simulink model "cst_robotarm_Identification"  (R2022b)
settings: Solver=ode23t  StartTime=0.0  StopTime=40  FixedStep=0.001  MaxStep=0.05  RelTol=1e-3  EnableMultiTasking=on
model workspace (MAT data in the model file):
  DCMotor_J = 0.0946866703633
  DCMotor_K = 0.477771340295
  DCMotor_Kf = 0.921434142151
  DCMotor_L = 0.000316454712175
  DCMotor_R = 4.99938152603
  Ts = 0.01
  dFilt = [1 -0.1202]
  nFilt = [0.4399 0.4399]
undefined symbols (not defined in the file or in its folder): sigbuilder_block, X, Y, Z
libraries: sm_lib x244, fl_lib x75, nesl_utility x28, ee_lib x21, simulink x6, slpidlib x6
(part 1 of 7)
settings Model: Creator=The MathWorks, Inc.  LastModifiedBy=Niki
settings SolverCC: AlgebraicLoopSolver=TrustRegion
settings DataIOCC: LimitDataPoints=on  SaveFormat=Array  InspectSignalLogs=on  SaveTime=off  ReturnWorkspaceOutputs=off
settings OptimizationCC: ExpressionDepthLimit=2147483647  LifeSpan=inf
settings DebuggingCC: UnderspecifiedInitializationDetection=Classic  MergeDetectMultiDrivingBlocksExec=none  FcnCallInpInsideContextMsg=warning  UnconnectedInputMsg=warning  UnconnectedOutputMsg=warning  UnconnectedLineMsg=warning  StateNameClashWarn=warning  SFUnexpectedBacktrackingDiag=warning  SFNoUnconditionalDefaultTransitionDiag=warning  SFExecutionAtInitializationDiag=none  SFMachineParentedDataDiag=warning  ArithmeticOperatorsInVariantConditions=warning
settings HardwareCC: ProdBitPerPointer=32  ProdBitPerSizeT=32  ProdBitPerPtrDiffT=32  ProdLargestAtomicFloat=None  ProdIntDivRoundTo=Undefined  ProdEndianess=Unspecified  ProdWordSize=32  ProdHWDeviceType=32-bit Generic
settings ModelReferenceCC: EnableRefExpFcnMdlSchedulingChecks=on  PropagateSignalLabelsOutOfModel=off
settings SFSimCC: SimUseLocalCustomCode=off  CustomCodeUndefinedFunction=UseInterfaceOnly
settings RTWCC: RTWUseLocalCustomCode=off
settings CodeAppCC: StateflowObjectComments=on
settings GRTTargetCC: TargetLangStandard=C89/C90 (ANSI)  CombineOutputUpdateFcns=off  GRTInterface=on
settings ConfigComp: CovMetricSettings=dw  CovSaveCumulativeToWorkspaceVar=on  CovSaveSingleToWorkspaceVar=on  CovExternalEMLEnable=off  CovSFcnEnable=off
settings SimscapeCC: SimscapeNormalizeSystem=off
settings ConfigurationSet: Description=SimMechanics 2G
settings DiagnosticsConfigSet: SimMechanicsUnconnectedFramePorts=none
settings ExplorerConfigSet: InternalSimMechanicsExplorerSettings="<ExplorerConfiguration><canonicalview>planar_xy</canonicalview><AnimationSetting><BasePlaybackSpeed>1.0</BasePlaybackSpeed><PlaybackSpeedFactor>1.0</PlaybackSpeedFactor></AnimationSetting><TilePanel><TileInfo><Tiles Columns=\"1\" Count=\"1\" Rows=\"1\"><Column Left=\"2\" Weight=\"1\"/><Column Left=\"708\"/><Row Top=\"2\" Weight=\"1\"/><Row Top=\"595\"/><Tile Height=\"1\" Width=\"1\" X=\"0\" Y=\"0\"/></Tiles></TileInfo><SceneInfo><SceneViewer><BGColor><R>0.80000001192092896</R><G>0.80000001192092896</G><B>0.80000001192092896</B></BGColor><Camera><Position><X>0.30752487944302698</X><Y>0.57922836563106395</Y><Z>0.35651305744246536</Z></Position><Center><X>-0.033772386749033274</X><Y>0.23793109943898419</Y><Z>0.015215791250393121</Z></Center><Up><X>-0.40824829046386307</X><Y>0.81649658092772615</Y><Z>-0.40824829046386307</Z></Up><Left>-0.063283674940751766</Left><Right>0.063283674940751766</Right><Bottom>-0.22321517040744418</Bottom><Top>0.22321517040744418</Top></Camera></SceneViewer></SceneInfo></TilePanel></ExplorerConfiguration>"

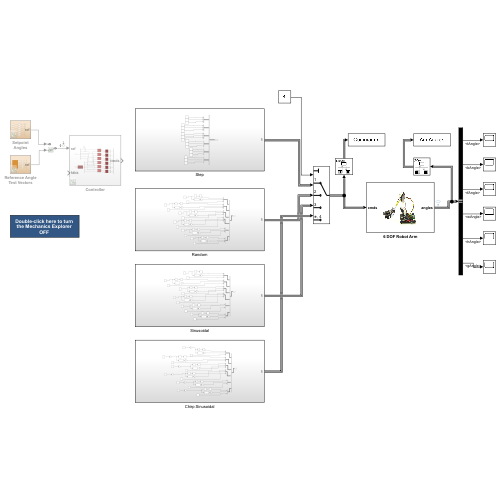
[thumbnail: Simulink's stored preview of the top-level diagram]
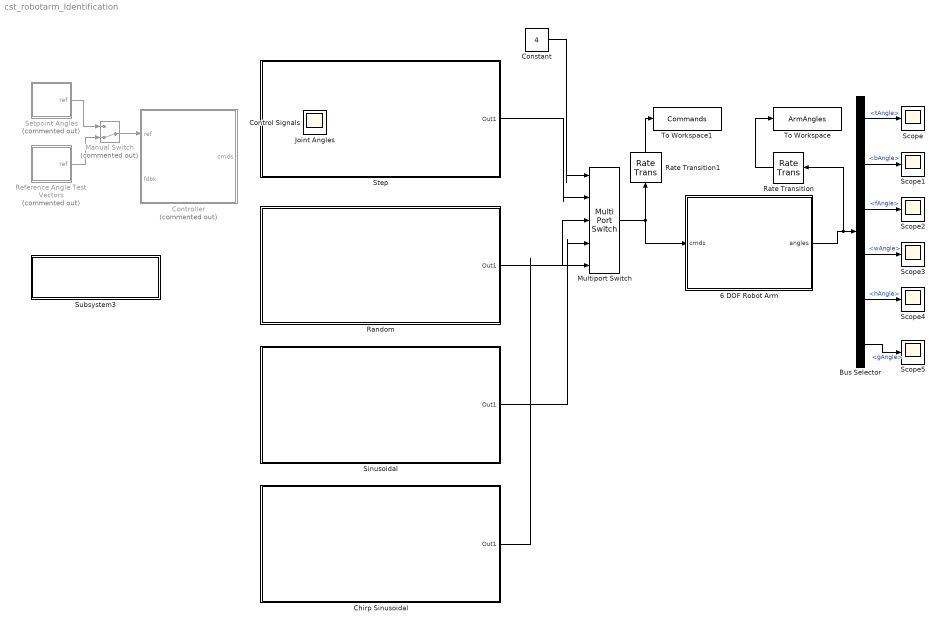
== system cst_robotarm_Identification ==
  6 DOF Robot Arm : Subsystem
      mask Display: image('RobotArmSystem.jpg',[0.2 0.05 0.6 0.9])
  Bus Selector : BusSelector  OutputSignals=tAngle,bAngle,fAngle,wAngle,hAngle,gAngle
  Chirp Sinusoidal : Subsystem
  Constant : Constant  Value=4
  Controller : Subsystem  Commented=on
  Manual Switch : ManualSwitch  Commented=on  CurrentSetting=0
  Multiport Switch : MultiPortSwitch  Inputs=4  SaturateOnIntegerOverflow=off  InputSameDT=off
  Random : Subsystem
  Rate Transition : RateTransition  OutPortSampleTime=0.01
  Rate Transition1 : RateTransition  OutPortSampleTime=0.01
  Reference Angle Test Vectors : Subsystem  Commented=on
  Scope{,1..5} (6 alike) : Scope
  Setpoint Angles : Subsystem  Commented=on
  Sinusoidal : Subsystem
  Step : Subsystem
  Subsystem3 : Subsystem
      mask init:
      | % Get current simulation mode
      | vizStatus = get_param(gcs,'SimMechanicsOpenEditorOnUpdate');
      | 
      | if strcmp(vizStatus,'on')
      |     viz = 'OFF';
      | else
      |     viz = 'ON';
      | end
      settings: OpenFcn=|
      | % Get current SimMechanics Explorer status
      | vizStatus = get_param(gcs ,'SimMechanicsOpenEditorOnUpdate');
      | 
      | if strcmp(vizStatus,'on')
      | % Set SimMechanics Explorer status to OFF
      |      set_param(gcs,'SimMechanicsOpenEditorOnUpdate','off');
      |      set_param(gcb,'BackgroundColor','[0.4706, 0.4706, 0.4706]');
      |      set_param(gcs,'SimulationCommand','update');
      | else
      | % Set SimMechanics Explorer status to ON
      |      set_param(gcs,'SimMechanicsOpenEditorOnUpdate','on');
      |      set_param(gcb,'BackgroundColor','[0.1961, 0.3412, 0.5176]')
      |      set_param(gcs,'SimulationCommand','update');
      | end
      mask Display:
      | color('white')
      | text(0.5,0.65,'Double-click here to turn\nthe Mechanics Explorer',...
      |     'horizontalAlignment','center',...
      |     'verticalAlignment','middle');
      | text(0.5,0.25,viz,...
      |     'horizontalAlignment','center',...
      |     'verticalAlignment','middle')
  To Workspace : ToWorkspace  VariableName=ArmAngles  SaveFormat=Structure With Time  SampleTime=-1
  To Workspace1 : ToWorkspace  VariableName=Commands  SaveFormat=Structure With Time  SampleTime=-1
  Control Signals : Scope
  Joint Angles : Scope
  wires:
  Manual Switch/1 -> Controller/1(ref)
  Reference Angle Test Vectors/1(ref) -> Manual Switch/2
  Setpoint Angles/1(ref) -> Manual Switch/1
  6 DOF Robot Arm/1(angles) -> Rate Transition/1, Bus Selector/1
  Bus Selector/1 -> Scope/1  "<tAngle>"
  Bus Selector/2 -> Scope1/1  "<bAngle>"
  Bus Selector/3 -> Scope2/1  "<fAngle>"
  Bus Selector/4 -> Scope3/1  "<wAngle>"
  Bus Selector/5 -> Scope4/1  "<hAngle>"
  Bus Selector/6 -> Scope5/1  "<gAngle>"
  Rate Transition/1 -> To Workspace/1
  Rate Transition1/1 -> To Workspace1/1
  Multiport Switch/1 -> 6 DOF Robot Arm/1(cmds), Rate Transition1/1
  Random/1(Out1) -> Multiport Switch/3
  Step/1(Out1) -> Multiport Switch/2
  Sinusoidal/1(Out1) -> Multiport Switch/4
  Constant/1 -> Multiport Switch/1
  Chirp Sinusoidal/1(Out1) -> Multiport Switch/5

== system cst_robotarm_Identification/6 DOF Robot Arm ==
  note: 6 DOF Robot Arm Manipulator - Electrical + Mechanical Plant Model
  cmds : Inport
  6 DOF Robot Arm Mechanics : Subsystem
      mask Display: image('RobotArm_Mechanics.jpg',[0.1 0 0.8 1])
  Bus Creator : BusCreator  Inputs=6
  Bus Selector : BusSelector  OutputSignals=tCMD,bCMD,fCMD,wCMD,hCMD,gCMD
  DC Motors : Subsystem
      mask Display: image('MultiServos.jpg',[0.25 0.1 0.5 0.8])
  PS-Simulink Converter{,1..5} (6 alike) : nesl_utility/PS-Simulink Converter  PhysicalDomain=network_engine_domain  SubClassName=ps_output  LeftPortType=input  RightPortType=output  PseudoPeriodic=off  Frequencies=[]  VectorFormat=1-D array  Unit=rad  AffineConversion=off
  angles : Outport  VectorParamsAs1DForOutWhenUnconnected=off
  wires:
  Bus Creator/1 -> angles/1
  PS-Simulink Converter2/1 -> Bus Creator/3  "fAngle"
  PS-Simulink Converter5/1 -> Bus Creator/6  "gAngle"
  PS-Simulink Converter/1 -> Bus Creator/1  "tAngle"
  PS-Simulink Converter1/1 -> Bus Creator/2  "bAngle"
  PS-Simulink Converter3/1 -> Bus Creator/4  "wAngle"
  PS-Simulink Converter4/1 -> Bus Creator/5  "hAngle"
  Bus Selector/6 -> DC Motors/6(gCMD)  "<gCMD>"
  Bus Selector/3 -> DC Motors/3(fCMD)  "<fCMD>"
  Bus Selector/4 -> DC Motors/4(wCMD)  "<wCMD>"
  Bus Selector/2 -> DC Motors/2(bCMD)  "<bCMD>"
  Bus Selector/5 -> DC Motors/5(hCMD)  "<hCMD>"
  Bus Selector/1 -> DC Motors/1(tCMD)  "<tCMD>"
  cmds/1 -> Bus Selector/1
  connections:
  PS-Simulink Converter2/LConn1 -- 6 DOF Robot Arm Mechanics/RConn3
  DC Motors/RConn7 -- 6 DOF Robot Arm Mechanics/LConn7
  DC Motors/RConn8 -- 6 DOF Robot Arm Mechanics/LConn8
  DC Motors/RConn6 -- 6 DOF Robot Arm Mechanics/LConn6
  PS-Simulink Converter/LConn1 -- 6 DOF Robot Arm Mechanics/RConn1
  DC Motors/RConn2 -- 6 DOF Robot Arm Mechanics/LConn2
  DC Motors/RConn5 -- 6 DOF Robot Arm Mechanics/LConn5
  DC Motors/RConn11 -- 6 DOF Robot Arm Mechanics/LConn11
  DC Motors/RConn12 -- 6 DOF Robot Arm Mechanics/LConn12
  DC Motors/RConn9 -- 6 DOF Robot Arm Mechanics/LConn9
  DC Motors/RConn3 -- 6 DOF Robot Arm Mechanics/LConn3
  DC Motors/RConn4 -- 6 DOF Robot Arm Mechanics/LConn4
  PS-Simulink Converter1/LConn1 -- 6 DOF Robot Arm Mechanics/RConn2
  PS-Simulink Converter4/LConn1 -- 6 DOF Robot Arm Mechanics/RConn5
  6 DOF Robot Arm Mechanics/RConn6 -- PS-Simulink Converter5/LConn1
  6 DOF Robot Arm Mechanics/RConn4 -- PS-Simulink Converter3/LConn1
  DC Motors/RConn10 -- 6 DOF Robot Arm Mechanics/LConn10
  DC Motors/RConn1 -- 6 DOF Robot Arm Mechanics/LConn1

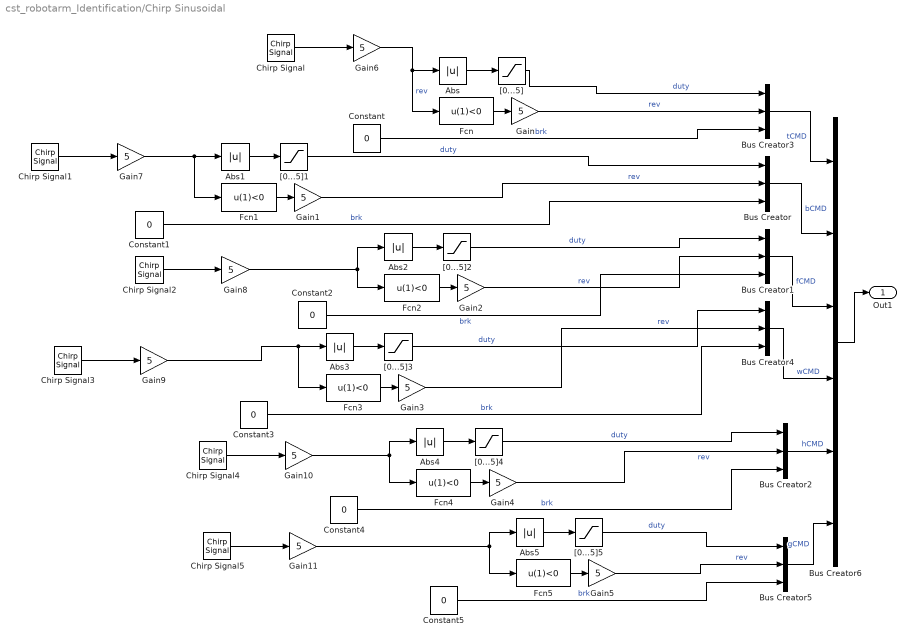
== system cst_robotarm_Identification/Chirp Sinusoidal ==
  Abs{,1..5} (6 alike) : Abs  SaturateOnIntegerOverflow=off
  Bus Creator{,1..5} (6 alike) : BusCreator  Inputs=3
  Bus Creator6 : BusCreator  Inputs=6
  Chirp Signal{,1..5} (6 alike) : simulink/Sources/Chirp Signal  f1=0.1  T=20  f2=2
  Constant{,1..5} (6 alike) : Constant  Value=0
  Fcn{,1..5} (6 alike) : Fcn  Expr=u(1)<0
  Gain{,1..11} (12 alike) : Gain  Gain=5
  [0...5]{,1..5} (6 alike) : Saturate  UpperLimit=5  LowerLimit=0
  Out1 : Outport
  wires:
  Fcn5/1 -> Gain5/1
  Gain11/1 -> Fcn5/1, Abs5/1
  Abs5/1 -> "[0...5]5"/1
  Fcn4/1 -> Gain4/1
  Gain10/1 -> Fcn4/1, Abs4/1
  Abs4/1 -> "[0...5]4"/1
  Fcn3/1 -> Gain3/1
  Gain9/1 -> Abs3/1, Fcn3/1
  Abs3/1 -> "[0...5]3"/1
  Fcn2/1 -> Gain2/1
  Gain8/1 -> Abs2/1, Fcn2/1
  Abs2/1 -> "[0...5]2"/1
  Gain7/1 -> Abs1/1, Fcn1/1
  Fcn1/1 -> Gain1/1
  Abs1/1 -> "[0...5]1"/1
  Abs/1 -> "[0...5]"/1
  Fcn/1 -> Gain/1
  Chirp Signal/1 -> Gain6/1
  Bus Creator6/1 -> Out1/1
  "[0...5]5"/1 -> Bus Creator5/1  "duty"
  Constant5/1 -> Bus Creator5/3  "brk"
  Bus Creator/1 -> Bus Creator6/2  "bCMD"
  Gain5/1 -> Bus Creator5/2  "rev"
  Bus Creator1/1 -> Bus Creator6/3  "fCMD"
  Constant3/1 -> Bus Creator4/3  "brk"
  Bus Creator5/1 -> Bus Creator6/6  "gCMD"
  Gain3/1 -> Bus Creator4/2  "rev"
  Bus Creator2/1 -> Bus Creator6/5  "hCMD"
  "[0...5]"/1 -> Bus Creator3/1  "duty"
  Bus Creator4/1 -> Bus Creator6/4  "wCMD"
  "[0...5]1"/1 -> Bus Creator/1  "duty"
  Constant1/1 -> Bus Creator/3  "brk"
  Gain1/1 -> Bus Creator/2  "rev"
  Gain2/1 -> Bus Creator1/2  "rev"
  Constant2/1 -> Bus Creator1/3  "brk"
  Constant/1 -> Bus Creator3/3  "brk"
  "[0...5]2"/1 -> Bus Creator1/1  "duty"
  Gain/1 -> Bus Creator3/2  "rev"
  Gain4/1 -> Bus Creator2/2  "rev"
  "[0...5]3"/1 -> Bus Creator4/1  "duty"
  Bus Creator3/1 -> Bus Creator6/1  "tCMD"
  "[0...5]4"/1 -> Bus Creator2/1  "duty"
  Constant4/1 -> Bus Creator2/3  "brk"
  Gain6/1 -> Abs/1, Fcn/1  "rev"
  Chirp Signal1/1 -> Gain7/1
  Chirp Signal2/1 -> Gain8/1
  Chirp Signal3/1 -> Gain9/1
  Chirp Signal4/1 -> Gain10/1
  Chirp Signal5/1 -> Gain11/1

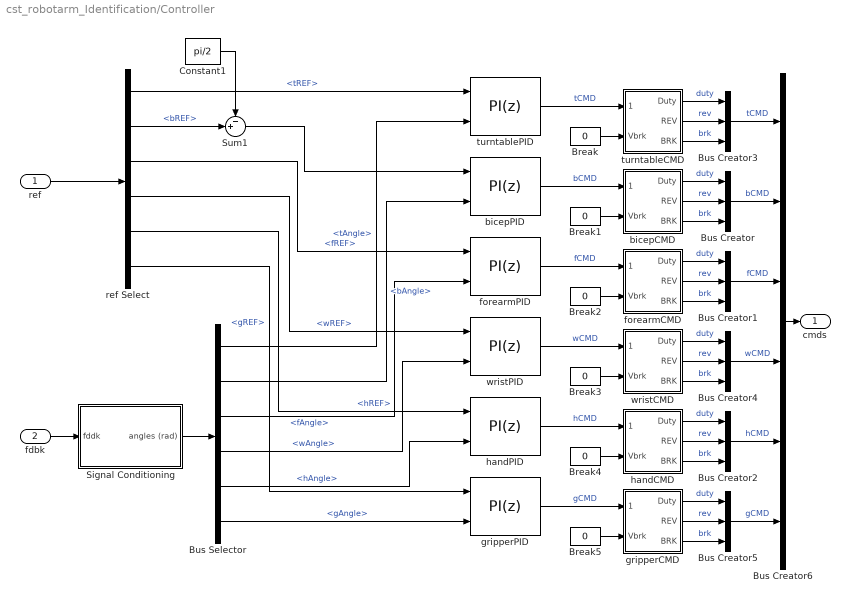
== system cst_robotarm_Identification/Controller ==
  ref : Inport
  fdbk : Inport  Port=2
  Break{,1..5} (6 alike) : Constant  Value=0
  Bus Creator{,1..5} (6 alike) : BusCreator  Inputs=3
  Bus Creator6 : BusCreator  Inputs=6
  Bus Selector : BusSelector  OutputSignals=tAngle,bAngle,fAngle,wAngle,hAngle,gAngle
  Constant1 : Constant  Value=pi/2
  Signal Conditioning : Subsystem
  Sum1 : Sum  Inputs=-+|
  bicepCMD : Subsystem
  bicepPID : slpidlib/PID Controller (2DOF)  Controller=PI  Form=Parallel  TimeDomain=Discrete-time  UseExternalTs=off  SampleTime=Ts  IntegratorMethod=Forward Euler  FilterMethod=Backward Euler  ControllerParametersSource=internal  P=17.1497999260389  I=18.7242369753632  UseKiTs=off  D=2.0  N=25  UseFilter=on  b=0.317016964341213  c=1  TunerSelectOption=Transfer Function Based (PID Tuner App)  InitialConditionSource=internal  InitialConditionForIntegrator=0  InitialConditionForFilter=0  DifferentiatorICPrevScaledInput=0  ExternalReset=none  TrackingMode=off  Kt=1  LimitOutput=on  SatLimitsSource=internal  UpperSaturationLimit=5  LowerSaturationLimit=-5  LinearizeAsGain=on  AntiWindupMode=clamping  Kb=1  LimitIntegrator=off  UpperIntegratorSaturationLimit=inf  LowerIntegratorSaturationLimit=-inf  POutMin=[]  POutMax=[]  IOutMin=[]  IOutMax=[]  DOutMin=[]  DOutMax=[]  NOutMin=[]  NOutMax=[]  bOutMin=[]  bOutMax=[]  cOutMin=[]  cOutMax=[]  SumOutMin=[]  SumOutMax=[]  SaturationOutMin=[]  SaturationOutMax=[]  PParamMin=[]  PParamMax=[]  IParamMin=[]  IParamMax=[]  DParamMin=[]  DParamMax=[]  NParamMin=[]  NParamMax=[]  bParamMin=[]  bParamMax=[]  cParamMin=[]  cParamMax=[]  KbParamMin=[]  KbParamMax=[]  KtParamMin=[]  KtParamMax=[]  KbOutMin=[]  KbOutMax=[]  KtOutMin=[]  KtOutMax=[]  IntegratorOutMin=[]  IntegratorOutMax=[]  FilterOutMin=[]  FilterOutMax=[]  SumI1OutMin=[]  SumI1OutMax=[]  SumI2OutMin=[]  SumI2OutMax=[]  SumI3OutMin=[]  SumI3OutMax=[]  SumI4OutMin=[]  SumI4OutMax=[]  SumDOutMin=[]  SumDOutMax=[]  Sum1OutMin=[]  Sum1OutMax=[]  Sum2OutMin=[]  Sum2OutMax=[]  Sum3OutMin=[]  Sum3OutMax=[]  DifferentiatorOutMin=[]  DifferentiatorOutMax=[]  FilterDiffOutCoefMin=[]  FilterDiffOutCoefMax=[]  ReciprocalOutMin=[]  ReciprocalOutMax=[]  SumDenOutMin=[]  SumDenOutMax=[]  SumNumOutMin=[]  SumNumOutMax=[]  DivideOutMin=[]  DivideOutMax=[]  UdiffTsProdOutMin=[]  UdiffTsProdOutMax=[]  NTsProdOutMin=[]  NTsProdOutMax=[]  UintegralTsProdOutMin=[]  UintegralTsProdOutMax=[]  UngainTsProdOutMin=[]  UngainTsProdOutMax=[]  ClampingZeroOutDataTypeStr=Inherit: Inherit via back propagation  ClampingZeroOutMin=[]  ClampingZeroOutMax=[]  FilterDenConstantOutDataTypeStr=Inherit: Inherit via back propagation  FilterDenConstantOutMin=[]  FilterDenConstantOutMax=[]  PCopyOutDataTypeStr=Inherit: Inherit via back propagation  PCopyOutMin=[]  PCopyOutMax=[]  NCopyOutDataTypeStr=Inherit: Inherit via back propagation  NCopyOutMin=[]  NCopyOutMax=[]  IntegratorContinuousStateAttributes=''  IntegratorStateMustResolveToSignalObject=off  IntegratorRTWStateStorageClass=Auto  FilterContinuousStateAttributes=''  FilterStateMustResolveToSignalObject=off  FilterRTWStateStorageClass=Auto  ParallelPVariant=InternalParameters  IdealPVariant=Disabled  IVariant=InternalParameters  DVariant=Disabled  bVariant=InternalParameters  cVariant=Disabled  IntegratorVariant=Discrete  SatVariant=Enabled  AWVariant=DiscClampingParallel  PCopyVariant=Disabled  TRVariant=Disabled  FdbkBlocksVariant=Forward  IdealPFdbkVariant=Disabled  SatFdbkVariant=Disabled  DerivativeFilterVariant=Disabled  NVariant=Disabled  NCopyVariant=Disabled_SignalSpec  FilterICVariant=Disabled  IntegratorICVariant=InternalICs  ExternalResetVariant=Disabled  TRSumVariant=Passthrough  SumFdbkVariant=Disabled  SumVariant=Sum_PI  TsampFilterVariant=InternalTs  TsampNgainVariant=Passthrough  TsampIntegralVariant=Passthrough  ExternalSaturationOutDataTypeStr=Inherit: Same as second input
  forearmCMD : Subsystem
  forearmPID : slpidlib/PID Controller (2DOF)  Controller=PI  Form=Parallel  TimeDomain=Discrete-time  UseExternalTs=off  SampleTime=Ts  IntegratorMethod=Forward Euler  FilterMethod=Backward Euler  ControllerParametersSource=internal  P=11.7551752480378  I=10.4523717996073  UseKiTs=off  D=2.0  N=25  UseFilter=on  b=0.528901562669871  c=1  TunerSelectOption=Transfer Function Based (PID Tuner App)  InitialConditionSource=internal  InitialConditionForIntegrator=0  InitialConditionForFilter=0  DifferentiatorICPrevScaledInput=0  ExternalReset=none  TrackingMode=off  Kt=1  LimitOutput=on  SatLimitsSource=internal  UpperSaturationLimit=5  LowerSaturationLimit=-5  LinearizeAsGain=on  AntiWindupMode=clamping  Kb=1  LimitIntegrator=off  UpperIntegratorSaturationLimit=inf  LowerIntegratorSaturationLimit=-inf  POutMin=[]  POutMax=[]  IOutMin=[]  IOutMax=[]  DOutMin=[]  DOutMax=[]  NOutMin=[]  NOutMax=[]  bOutMin=[]  bOutMax=[]  cOutMin=[]  cOutMax=[]  SumOutMin=[]  SumOutMax=[]  SaturationOutMin=[]  SaturationOutMax=[]  PParamMin=[]  PParamMax=[]  IParamMin=[]  IParamMax=[]  DParamMin=[]  DParamMax=[]  NParamMin=[]  NParamMax=[]  bParamMin=[]  bParamMax=[]  cParamMin=[]  cParamMax=[]  KbParamMin=[]  KbParamMax=[]  KtParamMin=[]  KtParamMax=[]  KbOutMin=[]  KbOutMax=[]  KtOutMin=[]  KtOutMax=[]  IntegratorOutMin=[]  IntegratorOutMax=[]  FilterOutMin=[]  FilterOutMax=[]  SumI1OutMin=[]  SumI1OutMax=[]  SumI2OutMin=[]  SumI2OutMax=[]  SumI3OutMin=[]  SumI3OutMax=[]  SumI4OutMin=[]  SumI4OutMax=[]  SumDOutMin=[]  SumDOutMax=[]  Sum1OutMin=[]  Sum1OutMax=[]  Sum2OutMin=[]  Sum2OutMax=[]  Sum3OutMin=[]  Sum3OutMax=[]  DifferentiatorOutMin=[]  DifferentiatorOutMax=[]  FilterDiffOutCoefMin=[]  FilterDiffOutCoefMax=[]  ReciprocalOutMin=[]  ReciprocalOutMax=[]  SumDenOutMin=[]  SumDenOutMax=[]  SumNumOutMin=[]  SumNumOutMax=[]  DivideOutMin=[]  DivideOutMax=[]  UdiffTsProdOutMin=[]  UdiffTsProdOutMax=[]  NTsProdOutMin=[]  NTsProdOutMax=[]  UintegralTsProdOutMin=[]  UintegralTsProdOutMax=[]  UngainTsProdOutMin=[]  UngainTsProdOutMax=[]  ClampingZeroOutDataTypeStr=Inherit: Inherit via back propagation  ClampingZeroOutMin=[]  ClampingZeroOutMax=[]  FilterDenConstantOutDataTypeStr=Inherit: Inherit via back propagation  FilterDenConstantOutMin=[]  FilterDenConstantOutMax=[]  PCopyOutDataTypeStr=Inherit: Inherit via back propagation  PCopyOutMin=[]  PCopyOutMax=[]  NCopyOutDataTypeStr=Inherit: Inherit via back propagation  NCopyOutMin=[]  NCopyOutMax=[]  IntegratorContinuousStateAttributes=''  IntegratorStateMustResolveToSignalObject=off  IntegratorRTWStateStorageClass=Auto  FilterContinuousStateAttributes=''  FilterStateMustResolveToSignalObject=off  FilterRTWStateStorageClass=Auto  ParallelPVariant=InternalParameters  IdealPVariant=Disabled  IVariant=InternalParameters  DVariant=Disabled  bVariant=InternalParameters  cVariant=Disabled  IntegratorVariant=Discrete  SatVariant=Enabled  AWVariant=DiscClampingParallel  PCopyVariant=Disabled  TRVariant=Disabled  FdbkBlocksVariant=Forward  IdealPFdbkVariant=Disabled  SatFdbkVariant=Disabled  DerivativeFilterVariant=Disabled  NVariant=Disabled  NCopyVariant=Disabled_SignalSpec  FilterICVariant=Disabled  IntegratorICVariant=InternalICs  ExternalResetVariant=Disabled  TRSumVariant=Passthrough  SumFdbkVariant=Disabled  SumVariant=Sum_PI  TsampFilterVariant=InternalTs  TsampNgainVariant=Passthrough  TsampIntegralVariant=Passthrough  ExternalSaturationOutDataTypeStr=Inherit: Same as second input
  gripperCMD : Subsystem
  gripperPID : slpidlib/PID Controller (2DOF)  Controller=PI  Form=Parallel  TimeDomain=Discrete-time  UseExternalTs=off  SampleTime=Ts  IntegratorMethod=Forward Euler  FilterMethod=Backward Euler  ControllerParametersSource=internal  P=11.8990340415483  I=10.4712956356752  UseKiTs=off  D=2.0  N=25  UseFilter=on  b=0.534221967296952  c=1  TunerSelectOption=Transfer Function Based (PID Tuner App)  InitialConditionSource=internal  InitialConditionForIntegrator=0  InitialConditionForFilter=0  DifferentiatorICPrevScaledInput=0  ExternalReset=none  TrackingMode=off  Kt=1  LimitOutput=on  SatLimitsSource=internal  UpperSaturationLimit=5  LowerSaturationLimit=-5  LinearizeAsGain=on  AntiWindupMode=clamping  Kb=1  LimitIntegrator=off  UpperIntegratorSaturationLimit=inf  LowerIntegratorSaturationLimit=-inf  POutMin=[]  POutMax=[]  IOutMin=[]  IOutMax=[]  DOutMin=[]  DOutMax=[]  NOutMin=[]  NOutMax=[]  bOutMin=[]  bOutMax=[]  cOutMin=[]  cOutMax=[]  SumOutMin=[]  SumOutMax=[]  SaturationOutMin=[]  SaturationOutMax=[]  PParamMin=[]  PParamMax=[]  IParamMin=[]  IParamMax=[]  DParamMin=[]  DParamMax=[]  NParamMin=[]  NParamMax=[]  bParamMin=[]  bParamMax=[]  cParamMin=[]  cParamMax=[]  KbParamMin=[]  KbParamMax=[]  KtParamMin=[]  KtParamMax=[]  KbOutMin=[]  KbOutMax=[]  KtOutMin=[]  KtOutMax=[]  IntegratorOutMin=[]  IntegratorOutMax=[]  FilterOutMin=[]  FilterOutMax=[]  SumI1OutMin=[]  SumI1OutMax=[]  SumI2OutMin=[]  SumI2OutMax=[]  SumI3OutMin=[]  SumI3OutMax=[]  SumI4OutMin=[]  SumI4OutMax=[]  SumDOutMin=[]  SumDOutMax=[]  Sum1OutMin=[]  Sum1OutMax=[]  Sum2OutMin=[]  Sum2OutMax=[]  Sum3OutMin=[]  Sum3OutMax=[]  DifferentiatorOutMin=[]  DifferentiatorOutMax=[]  FilterDiffOutCoefMin=[]  FilterDiffOutCoefMax=[]  ReciprocalOutMin=[]  ReciprocalOutMax=[]  SumDenOutMin=[]  SumDenOutMax=[]  SumNumOutMin=[]  SumNumOutMax=[]  DivideOutMin=[]  DivideOutMax=[]  UdiffTsProdOutMin=[]  UdiffTsProdOutMax=[]  NTsProdOutMin=[]  NTsProdOutMax=[]  UintegralTsProdOutMin=[]  UintegralTsProdOutMax=[]  UngainTsProdOutMin=[]  UngainTsProdOutMax=[]  ClampingZeroOutDataTypeStr=Inherit: Inherit via back propagation  ClampingZeroOutMin=[]  ClampingZeroOutMax=[]  FilterDenConstantOutDataTypeStr=Inherit: Inherit via back propagation  FilterDenConstantOutMin=[]  FilterDenConstantOutMax=[]  PCopyOutDataTypeStr=Inherit: Inherit via back propagation  PCopyOutMin=[]  PCopyOutMax=[]  NCopyOutDataTypeStr=Inherit: Inherit via back propagation  NCopyOutMin=[]  NCopyOutMax=[]  IntegratorContinuousStateAttributes=''  IntegratorStateMustResolveToSignalObject=off  IntegratorRTWStateStorageClass=Auto  FilterContinuousStateAttributes=''  FilterStateMustResolveToSignalObject=off  FilterRTWStateStorageClass=Auto  ParallelPVariant=InternalParameters  IdealPVariant=Disabled  IVariant=InternalParameters  DVariant=Disabled  bVariant=InternalParameters  cVariant=Disabled  IntegratorVariant=Discrete  SatVariant=Enabled  AWVariant=DiscClampingParallel  PCopyVariant=Disabled  TRVariant=Disabled  FdbkBlocksVariant=Forward  IdealPFdbkVariant=Disabled  SatFdbkVariant=Disabled  DerivativeFilterVariant=Disabled  NVariant=Disabled  NCopyVariant=Disabled_SignalSpec  FilterICVariant=Disabled  IntegratorICVariant=InternalICs  ExternalResetVariant=Disabled  TRSumVariant=Passthrough  SumFdbkVariant=Disabled  SumVariant=Sum_PI  TsampFilterVariant=InternalTs  TsampNgainVariant=Passthrough  TsampIntegralVariant=Passthrough  ExternalSaturationOutDataTypeStr=Inherit: Same as second input
  handCMD : Subsystem
  handPID : slpidlib/PID Controller (2DOF)  Controller=PI  Form=Parallel  TimeDomain=Discrete-time  UseExternalTs=off  SampleTime=Ts  IntegratorMethod=Forward Euler  FilterMethod=Backward Euler  ControllerParametersSource=internal  P=11.2816850078634  I=9.22879347051619  UseKiTs=off  D=2.0  N=25  UseFilter=on  b=0.566281521673299  c=1  TunerSelectOption=Transfer Function Based (PID Tuner App)  InitialConditionSource=internal  InitialConditionForIntegrator=0  InitialConditionForFilter=0  DifferentiatorICPrevScaledInput=0  ExternalReset=none  TrackingMode=off  Kt=1  LimitOutput=on  SatLimitsSource=internal  UpperSaturationLimit=5  LowerSaturationLimit=-5  LinearizeAsGain=on  AntiWindupMode=clamping  Kb=1  LimitIntegrator=off  UpperIntegratorSaturationLimit=inf  LowerIntegratorSaturationLimit=-inf  POutMin=[]  POutMax=[]  IOutMin=[]  IOutMax=[]  DOutMin=[]  DOutMax=[]  NOutMin=[]  NOutMax=[]  bOutMin=[]  bOutMax=[]  cOutMin=[]  cOutMax=[]  SumOutMin=[]  SumOutMax=[]  SaturationOutMin=[]  SaturationOutMax=[]  PParamMin=[]  PParamMax=[]  IParamMin=[]  IParamMax=[]  DParamMin=[]  DParamMax=[]  NParamMin=[]  NParamMax=[]  bParamMin=[]  bParamMax=[]  cParamMin=[]  cParamMax=[]  KbParamMin=[]  KbParamMax=[]  KtParamMin=[]  KtParamMax=[]  KbOutMin=[]  KbOutMax=[]  KtOutMin=[]  KtOutMax=[]  IntegratorOutMin=[]  IntegratorOutMax=[]  FilterOutMin=[]  FilterOutMax=[]  SumI1OutMin=[]  SumI1OutMax=[]  SumI2OutMin=[]  SumI2OutMax=[]  SumI3OutMin=[]  SumI3OutMax=[]  SumI4OutMin=[]  SumI4OutMax=[]  SumDOutMin=[]  SumDOutMax=[]  Sum1OutMin=[]  Sum1OutMax=[]  Sum2OutMin=[]  Sum2OutMax=[]  Sum3OutMin=[]  Sum3OutMax=[]  DifferentiatorOutMin=[]  DifferentiatorOutMax=[]  FilterDiffOutCoefMin=[]  FilterDiffOutCoefMax=[]  ReciprocalOutMin=[]  ReciprocalOutMax=[]  SumDenOutMin=[]  SumDenOutMax=[]  SumNumOutMin=[]  SumNumOutMax=[]  DivideOutMin=[]  DivideOutMax=[]  UdiffTsProdOutMin=[]  UdiffTsProdOutMax=[]  NTsProdOutMin=[]  NTsProdOutMax=[]  UintegralTsProdOutMin=[]  UintegralTsProdOutMax=[]  UngainTsProdOutMin=[]  UngainTsProdOutMax=[]  ClampingZeroOutDataTypeStr=Inherit: Inherit via back propagation  ClampingZeroOutMin=[]  ClampingZeroOutMax=[]  FilterDenConstantOutDataTypeStr=Inherit: Inherit via back propagation  FilterDenConstantOutMin=[]  FilterDenConstantOutMax=[]  PCopyOutDataTypeStr=Inherit: Inherit via back propagation  PCopyOutMin=[]  PCopyOutMax=[]  NCopyOutDataTypeStr=Inherit: Inherit via back propagation  NCopyOutMin=[]  NCopyOutMax=[]  IntegratorContinuousStateAttributes=''  IntegratorStateMustResolveToSignalObject=off  IntegratorRTWStateStorageClass=Auto  FilterContinuousStateAttributes=''  FilterStateMustResolveToSignalObject=off  FilterRTWStateStorageClass=Auto  ParallelPVariant=InternalParameters  IdealPVariant=Disabled  IVariant=InternalParameters  DVariant=Disabled  bVariant=InternalParameters  cVariant=Disabled  IntegratorVariant=Discrete  SatVariant=Enabled  AWVariant=DiscClampingParallel  PCopyVariant=Disabled  TRVariant=Disabled  FdbkBlocksVariant=Forward  IdealPFdbkVariant=Disabled  SatFdbkVariant=Disabled  DerivativeFilterVariant=Disabled  NVariant=Disabled  NCopyVariant=Disabled_SignalSpec  FilterICVariant=Disabled  IntegratorICVariant=InternalICs  ExternalResetVariant=Disabled  TRSumVariant=Passthrough  SumFdbkVariant=Disabled  SumVariant=Sum_PI  TsampFilterVariant=InternalTs  TsampNgainVariant=Passthrough  TsampIntegralVariant=Passthrough  ExternalSaturationOutDataTypeStr=Inherit: Same as second input
  ref Select : BusSelector  OutputSignals=tREF,bREF,fREF,wREF,hREF,gREF
  turntableCMD : Subsystem
  turntablePID : slpidlib/PID Controller (2DOF)  Controller=PI  Form=Parallel  TimeDomain=Discrete-time  UseExternalTs=off  SampleTime=Ts  IntegratorMethod=Forward Euler  FilterMethod=Backward Euler  ControllerParametersSource=internal  P=11.2307078727746  I=9.22773156440348  UseKiTs=off  D=2.0  N=25  UseFilter=on  b=0.564830483665764  c=1  TunerSelectOption=Transfer Function Based (PID Tuner App)  InitialConditionSource=internal  InitialConditionForIntegrator=0  InitialConditionForFilter=0  DifferentiatorICPrevScaledInput=0  ExternalReset=none  TrackingMode=off  Kt=1  LimitOutput=on  SatLimitsSource=internal  UpperSaturationLimit=5  LowerSaturationLimit=-5  LinearizeAsGain=on  AntiWindupMode=clamping  Kb=1  LimitIntegrator=off  UpperIntegratorSaturationLimit=inf  LowerIntegratorSaturationLimit=-inf  POutMin=[]  POutMax=[]  IOutMin=[]  IOutMax=[]  DOutMin=[]  DOutMax=[]  NOutMin=[]  NOutMax=[]  bOutMin=[]  bOutMax=[]  cOutMin=[]  cOutMax=[]  SumOutMin=[]  SumOutMax=[]  SaturationOutMin=[]  SaturationOutMax=[]  PParamMin=[]  PParamMax=[]  IParamMin=[]  IParamMax=[]  DParamMin=[]  DParamMax=[]  NParamMin=[]  NParamMax=[]  bParamMin=[]  bParamMax=[]  cParamMin=[]  cParamMax=[]  KbParamMin=[]  KbParamMax=[]  KtParamMin=[]  KtParamMax=[]  KbOutMin=[]  KbOutMax=[]  KtOutMin=[]  KtOutMax=[]  IntegratorOutMin=[]  IntegratorOutMax=[]  FilterOutMin=[]  FilterOutMax=[]  SumI1OutMin=[]  SumI1OutMax=[]  SumI2OutMin=[]  SumI2OutMax=[]  SumI3OutMin=[]  SumI3OutMax=[]  SumI4OutMin=[]  SumI4OutMax=[]  SumDOutMin=[]  SumDOutMax=[]  Sum1OutMin=[]  Sum1OutMax=[]  Sum2OutMin=[]  Sum2OutMax=[]  Sum3OutMin=[]  Sum3OutMax=[]  DifferentiatorOutMin=[]  DifferentiatorOutMax=[]  FilterDiffOutCoefMin=[]  FilterDiffOutCoefMax=[]  ReciprocalOutMin=[]  ReciprocalOutMax=[]  SumDenOutMin=[]  SumDenOutMax=[]  SumNumOutMin=[]  SumNumOutMax=[]  DivideOutMin=[]  DivideOutMax=[]  UdiffTsProdOutMin=[]  UdiffTsProdOutMax=[]  NTsProdOutMin=[]  NTsProdOutMax=[]  UintegralTsProdOutMin=[]  UintegralTsProdOutMax=[]  UngainTsProdOutMin=[]  UngainTsProdOutMax=[]  ClampingZeroOutDataTypeStr=Inherit: Inherit via back propagation  ClampingZeroOutMin=[]  ClampingZeroOutMax=[]  FilterDenConstantOutDataTypeStr=Inherit: Inherit via back propagation  FilterDenConstantOutMin=[]  FilterDenConstantOutMax=[]  PCopyOutDataTypeStr=Inherit: Inherit via back propagation  PCopyOutMin=[]  PCopyOutMax=[]  NCopyOutDataTypeStr=Inherit: Inherit via back propagation  NCopyOutMin=[]  NCopyOutMax=[]  IntegratorContinuousStateAttributes=''  IntegratorStateMustResolveToSignalObject=off  IntegratorRTWStateStorageClass=Auto  FilterContinuousStateAttributes=''  FilterStateMustResolveToSignalObject=off  FilterRTWStateStorageClass=Auto  ParallelPVariant=InternalParameters  IdealPVariant=Disabled  IVariant=InternalParameters  DVariant=Disabled  bVariant=InternalParameters  cVariant=Disabled  IntegratorVariant=Discrete  SatVariant=Enabled  AWVariant=DiscClampingParallel  PCopyVariant=Disabled  TRVariant=Disabled  FdbkBlocksVariant=Forward  IdealPFdbkVariant=Disabled  SatFdbkVariant=Disabled  DerivativeFilterVariant=Disabled  NVariant=Disabled  NCopyVariant=Disabled_SignalSpec  FilterICVariant=Disabled  IntegratorICVariant=InternalICs  ExternalResetVariant=Disabled  TRSumVariant=Passthrough  SumFdbkVariant=Disabled  SumVariant=Sum_PI  TsampFilterVariant=InternalTs  TsampNgainVariant=Passthrough  TsampIntegralVariant=Passthrough  ExternalSaturationOutDataTypeStr=Inherit: Same as second input
  wristCMD : Subsystem
  wristPID : slpidlib/PID Controller (2DOF)  Controller=PI  Form=Parallel  TimeDomain=Discrete-time  UseExternalTs=off  SampleTime=Ts  IntegratorMethod=Forward Euler  FilterMethod=Backward Euler  ControllerParametersSource=internal  P=12.3822622694296  I=11.6489143861249  UseKiTs=off  D=2.0  N=25  UseFilter=on  b=0.503586166878936  c=1  TunerSelectOption=Transfer Function Based (PID Tuner App)  InitialConditionSource=internal  InitialConditionForIntegrator=0  InitialConditionForFilter=0  DifferentiatorICPrevScaledInput=0  ExternalReset=none  TrackingMode=off  Kt=1  LimitOutput=on  SatLimitsSource=internal  UpperSaturationLimit=5  LowerSaturationLimit=-5  LinearizeAsGain=on  AntiWindupMode=clamping  Kb=1  LimitIntegrator=off  UpperIntegratorSaturationLimit=inf  LowerIntegratorSaturationLimit=-inf  POutMin=[]  POutMax=[]  IOutMin=[]  IOutMax=[]  DOutMin=[]  DOutMax=[]  NOutMin=[]  NOutMax=[]  bOutMin=[]  bOutMax=[]  cOutMin=[]  cOutMax=[]  SumOutMin=[]  SumOutMax=[]  SaturationOutMin=[]  SaturationOutMax=[]  PParamMin=[]  PParamMax=[]  IParamMin=[]  IParamMax=[]  DParamMin=[]  DParamMax=[]  NParamMin=[]  NParamMax=[]  bParamMin=[]  bParamMax=[]  cParamMin=[]  cParamMax=[]  KbParamMin=[]  KbParamMax=[]  KtParamMin=[]  KtParamMax=[]  KbOutMin=[]  KbOutMax=[]  KtOutMin=[]  KtOutMax=[]  IntegratorOutMin=[]  IntegratorOutMax=[]  FilterOutMin=[]  FilterOutMax=[]  SumI1OutMin=[]  SumI1OutMax=[]  SumI2OutMin=[]  SumI2OutMax=[]  SumI3OutMin=[]  SumI3OutMax=[]  SumI4OutMin=[]  SumI4OutMax=[]  SumDOutMin=[]  SumDOutMax=[]  Sum1OutMin=[]  Sum1OutMax=[]  Sum2OutMin=[]  Sum2OutMax=[]  Sum3OutMin=[]  Sum3OutMax=[]  DifferentiatorOutMin=[]  DifferentiatorOutMax=[]  FilterDiffOutCoefMin=[]  FilterDiffOutCoefMax=[]  ReciprocalOutMin=[]  ReciprocalOutMax=[]  SumDenOutMin=[]  SumDenOutMax=[]  SumNumOutMin=[]  SumNumOutMax=[]  DivideOutMin=[]  DivideOutMax=[]  UdiffTsProdOutMin=[]  UdiffTsProdOutMax=[]  NTsProdOutMin=[]  NTsProdOutMax=[]  UintegralTsProdOutMin=[]  UintegralTsProdOutMax=[]  UngainTsProdOutMin=[]  UngainTsProdOutMax=[]  ClampingZeroOutDataTypeStr=Inherit: Inherit via back propagation  ClampingZeroOutMin=[]  ClampingZeroOutMax=[]  FilterDenConstantOutDataTypeStr=Inherit: Inherit via back propagation  FilterDenConstantOutMin=[]  FilterDenConstantOutMax=[]  PCopyOutDataTypeStr=Inherit: Inherit via back propagation  PCopyOutMin=[]  PCopyOutMax=[]  NCopyOutDataTypeStr=Inherit: Inherit via back propagation  NCopyOutMin=[]  NCopyOutMax=[]  IntegratorContinuousStateAttributes=''  IntegratorStateMustResolveToSignalObject=off  IntegratorRTWStateStorageClass=Auto  FilterContinuousStateAttributes=''  FilterStateMustResolveToSignalObject=off  FilterRTWStateStorageClass=Auto  ParallelPVariant=InternalParameters  IdealPVariant=Disabled  IVariant=InternalParameters  DVariant=Disabled  bVariant=InternalParameters  cVariant=Disabled  IntegratorVariant=Discrete  SatVariant=Enabled  AWVariant=DiscClampingParallel  PCopyVariant=Disabled  TRVariant=Disabled  FdbkBlocksVariant=Forward  IdealPFdbkVariant=Disabled  SatFdbkVariant=Disabled  DerivativeFilterVariant=Disabled  NVariant=Disabled  NCopyVariant=Disabled_SignalSpec  FilterICVariant=Disabled  IntegratorICVariant=InternalICs  ExternalResetVariant=Disabled  TRSumVariant=Passthrough  SumFdbkVariant=Disabled  SumVariant=Sum_PI  TsampFilterVariant=InternalTs  TsampNgainVariant=Passthrough  TsampIntegralVariant=Passthrough  ExternalSaturationOutDataTypeStr=Inherit: Same as second input
  cmds : Outport  VectorParamsAs1DForOutWhenUnconnected=off
  wires:
  bicepCMD/1(Duty) -> Bus Creator/1  "duty"
  bicepCMD/2(REV) -> Bus Creator/2  "rev"
  bicepCMD/3(BRK) -> Bus Creator/3  "brk"
  forearmCMD/1(Duty) -> Bus Creator1/1  "duty"
  forearmCMD/2(REV) -> Bus Creator1/2  "rev"
  forearmCMD/3(BRK) -> Bus Creator1/3  "brk"
  handCMD/2(REV) -> Bus Creator2/2  "rev"
  handCMD/3(BRK) -> Bus Creator2/3  "brk"
  handCMD/1(Duty) -> Bus Creator2/1  "duty"
  bicepPID/1 -> bicepCMD/1(Vcmd)  "bCMD"
  Break1/1 -> bicepCMD/2(Vbrk)
  forearmPID/1 -> forearmCMD/1(Vcmd)  "fCMD"
  Break2/1 -> forearmCMD/2(Vbrk)
  handPID/1 -> handCMD/1(Vcmd)  "hCMD"
  Break4/1 -> handCMD/2(Vbrk)
  Bus Creator1/1 -> Bus Creator6/3  "fCMD"
  Bus Creator2/1 -> Bus Creator6/5  "hCMD"
  ref/1 -> ref Select/1
  turntableCMD/1(Duty) -> Bus Creator3/1  "duty"
  turntableCMD/2(REV) -> Bus Creator3/2  "rev"
  turntableCMD/3(BRK) -> Bus Creator3/3  "brk"
  turntablePID/1 -> turntableCMD/1(Vcmd)  "tCMD"
  Break/1 -> turntableCMD/2(Vbrk)
  Bus Creator3/1 -> Bus Creator6/1  "tCMD"
  wristCMD/2(REV) -> Bus Creator4/2  "rev"
  wristCMD/3(BRK) -> Bus Creator4/3  "brk"
  wristCMD/1(Duty) -> Bus Creator4/1  "duty"
  wristPID/1 -> wristCMD/1(Vcmd)  "wCMD"
  Break3/1 -> wristCMD/2(Vbrk)
  Bus Creator4/1 -> Bus Creator6/4  "wCMD"
  gripperCMD/2(REV) -> Bus Creator5/2  "rev"
  gripperCMD/3(BRK) -> Bus Creator5/3  "brk"
  gripperCMD/1(Duty) -> Bus Creator5/1  "duty"
  gripperPID/1 -> gripperCMD/1(Vcmd)  "gCMD"
  Break5/1 -> gripperCMD/2(Vbrk)
  Bus Creator5/1 -> Bus Creator6/6  "gCMD"
  Bus Creator/1 -> Bus Creator6/2  "bCMD"
  Bus Creator6/1 -> cmds/1
  Bus Selector/6 -> gripperPID/2  "<gAngle>"
  Bus Selector/5 -> handPID/2  "<hAngle>"
  Bus Selector/4 -> wristPID/2  "<wAngle>"
  Bus Selector/3 -> forearmPID/2  "<fAngle>"
  Bus Selector/1 -> turntablePID/2  "<tAngle>"
  ref Select/1 -> turntablePID/1  "<tREF>"
  ref Select/3 -> forearmPID/1  "<fREF>"
  ref Select/4 -> wristPID/1  "<wREF>"
  ref Select/5 -> handPID/1  "<hREF>"
  ref Select/6 -> gripperPID/1  "<gREF>"
  fdbk/1 -> Signal Conditioning/1(fddk)
  Signal Conditioning/1(angles (rad)) -> Bus Selector/1
  Sum1/1 -> bicepPID/1
  ref Select/2 -> Sum1/2  "<bREF>"
  Constant1/1 -> Sum1/1
  Bus Selector/2 -> bicepPID/2  "<bAngle>"

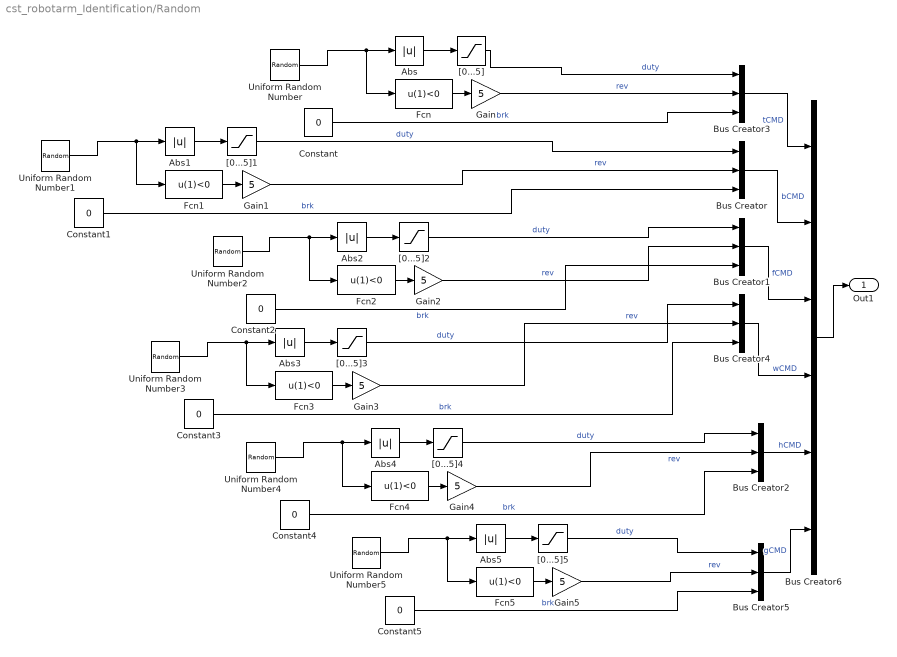
== system cst_robotarm_Identification/Random ==
  Abs{,1..5} (6 alike) : Abs  SaturateOnIntegerOverflow=off
  Bus Creator{,1..5} (6 alike) : BusCreator  Inputs=3
  Bus Creator6 : BusCreator  Inputs=6
  Constant{,1..5} (6 alike) : Constant  Value=0
  Fcn{,1..5} (6 alike) : Fcn  Expr=u(1)<0
  Gain{,1..5} (6 alike) : Gain  Gain=5
  Uniform Random Number{,1..5} (6 alike) : UniformRandomNumber  Minimum=-5  Maximum=5  SampleTime=0.01
  [0...5]{,1..5} (6 alike) : Saturate  UpperLimit=5  LowerLimit=0
  Out1 : Outport
  wires:
  Constant4/1 -> Bus Creator2/3  "brk"
  "[0...5]4"/1 -> Bus Creator2/1  "duty"
  Bus Creator3/1 -> Bus Creator6/1  "tCMD"
  "[0...5]3"/1 -> Bus Creator4/1  "duty"
  Gain4/1 -> Bus Creator2/2  "rev"
  Gain/1 -> Bus Creator3/2  "rev"
  "[0...5]2"/1 -> Bus Creator1/1  "duty"
  Constant/1 -> Bus Creator3/3  "brk"
  Constant2/1 -> Bus Creator1/3  "brk"
  Gain2/1 -> Bus Creator1/2  "rev"
  Gain1/1 -> Bus Creator/2  "rev"
  Constant1/1 -> Bus Creator/3  "brk"
  "[0...5]1"/1 -> Bus Creator/1  "duty"
  Bus Creator4/1 -> Bus Creator6/4  "wCMD"
  "[0...5]"/1 -> Bus Creator3/1  "duty"
  Bus Creator2/1 -> Bus Creator6/5  "hCMD"
  Gain3/1 -> Bus Creator4/2  "rev"
  Bus Creator5/1 -> Bus Creator6/6  "gCMD"
  Constant3/1 -> Bus Creator4/3  "brk"
  Bus Creator1/1 -> Bus Creator6/3  "fCMD"
  Gain5/1 -> Bus Creator5/2  "rev"
  Bus Creator/1 -> Bus Creator6/2  "bCMD"
  Constant5/1 -> Bus Creator5/3  "brk"
  "[0...5]5"/1 -> Bus Creator5/1  "duty"
  Bus Creator6/1 -> Out1/1
  Uniform Random Number/1 -> Fcn/1, Abs/1
  Fcn/1 -> Gain/1
  Abs/1 -> "[0...5]"/1
  Abs1/1 -> "[0...5]1"/1
  Fcn1/1 -> Gain1/1
  Uniform Random Number1/1 -> Fcn1/1, Abs1/1
  Abs2/1 -> "[0...5]2"/1
  Uniform Random Number2/1 -> Fcn2/1, Abs2/1
  Fcn2/1 -> Gain2/1
  Abs3/1 -> "[0...5]3"/1
  Uniform Random Number3/1 -> Fcn3/1, Abs3/1
  Fcn3/1 -> Gain3/1
  Abs4/1 -> "[0...5]4"/1
  Uniform Random Number4/1 -> Fcn4/1, Abs4/1
  Fcn4/1 -> Gain4/1
  Abs5/1 -> "[0...5]5"/1
  Uniform Random Number5/1 -> Fcn5/1, Abs5/1
  Fcn5/1 -> Gain5/1

== system cst_robotarm_Identification/Reference Angle Test Vectors ==
  Bus Creator : BusCreator  Inputs=6
  Gain{,1..5} (6 alike) : Gain  Gain=pi/180
  Joint Angle Test Vectors : Subsystem  Tag=STV Subsys  LoadFcn=sigbuilder_block('load');  StartFcn=sigbuilder_block('start');  StopFcn=sigbuilder_block('stop');  ClipboardFcn=sigbuilder_block('clipboard');  mask(Sigbuilder block){tuvar=[0:10]}
      mask help: Create and generate interchangeable groups of signals whose waveforms are piecewise linear.
      mask init:
      | if ~strcmp(get_param(bdroot(gcbh),'SimulationStatus'),'stopped') tuvar = sigbuilder_block('maskInit'); end
      settings: CopyFcn=sigbuilder_block('copy');  DeleteFcn=sigbuilder_block('delete');  ModelCloseFcn=sigbuilder_block('modelClose');  PreSaveFcn=sigbuilder_block('preSave');  PauseFcn=sigbuilder_block('pause')  ContinueFcn=sigbuilder_block('continue')  NameChangeFcn=sigbuilder_block('namechange');  OpenFcn=sigbuilder_block('open',[87 192 547 478.5 ]);  CloseFcn=sigbuilder_block('close');
      mask Display: plot(0, 0, 100, 100,[2, 2, 32, 32, 2], [68, 8, 8, 68, 68],[32, 2], [38, 38], [32, 19, 2],[53, 60, 44], [32, 17, 17, 2],[16, 16, 31, 31]);txt = getActiveGroup(gcbh);text(2, 100, txt,'verticalAlignment', 'top');
  ref : Outport  VectorParamsAs1DForOutWhenUnconnected=off
  wires:
  Joint Angle Test Vectors/1(Turntable Angle (deg)) -> Gain/1
  Joint Angle Test Vectors/2(Bicep Angle (deg)) -> Gain1/1
  Joint Angle Test Vectors/3(Forearm Angle (deg)) -> Gain2/1
  Joint Angle Test Vectors/4(Wrist Angle (deg)) -> Gain3/1
  Joint Angle Test Vectors/5(Hand Angle (deg)) -> Gain4/1
  Joint Angle Test Vectors/6(Gripper Angle (deg)) -> Gain5/1
  Bus Creator/1 -> ref/1
  Gain/1 -> Bus Creator/1  "tREF"
  Gain1/1 -> Bus Creator/2  "bREF"
  Gain2/1 -> Bus Creator/3  "fREF"
  Gain3/1 -> Bus Creator/4  "wREF"
  Gain4/1 -> Bus Creator/5  "hREF"
  Gain5/1 -> Bus Creator/6  "gREF"

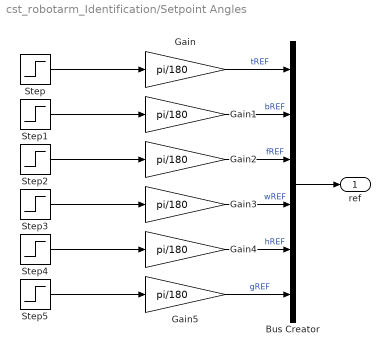
== system cst_robotarm_Identification/Setpoint Angles ==
  Bus Creator : BusCreator  Inputs=6
  Gain{,1..5} (6 alike) : Gain  Gain=pi/180
  Step : Step  Time=0  After=60  SampleTime=Ts
  Step1 : Step  Time=0  Before=90  After=80  SampleTime=Ts
  Step2 : Step  Time=0  After=60  SampleTime=Ts
  Step3 : Step  Time=0  After=90  SampleTime=Ts
  Step4 : Step  Time=0  After=90  SampleTime=Ts
  Step5 : Step  Time=0  After=30  SampleTime=Ts
  ref : Outport  VectorParamsAs1DForOutWhenUnconnected=off
  wires:
  Gain5/1 -> Bus Creator/6  "gREF"
  Gain4/1 -> Bus Creator/5  "hREF"
  Gain3/1 -> Bus Creator/4  "wREF"
  Gain2/1 -> Bus Creator/3  "fREF"
  Gain1/1 -> Bus Creator/2  "bREF"
  Gain/1 -> Bus Creator/1  "tREF"
  Bus Creator/1 -> ref/1
  Step/1 -> Gain/1
  Step1/1 -> Gain1/1
  Step2/1 -> Gain2/1
  Step3/1 -> Gain3/1
  Step4/1 -> Gain4/1
  Step5/1 -> Gain5/1

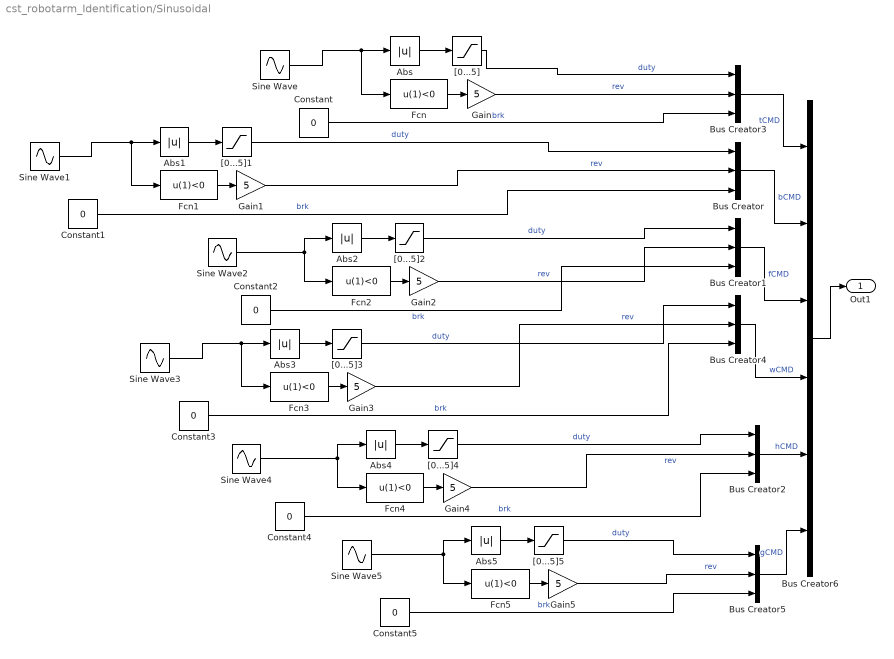
== system cst_robotarm_Identification/Sinusoidal ==
  Abs{,1..5} (6 alike) : Abs  SaturateOnIntegerOverflow=off
  Bus Creator{,1..5} (6 alike) : BusCreator  Inputs=3
  Bus Creator6 : BusCreator  Inputs=6
  Constant{,1..5} (6 alike) : Constant  Value=0
  Fcn{,1..5} (6 alike) : Fcn  Expr=u(1)<0
  Gain{,1..5} (6 alike) : Gain  Gain=5
  Sine Wave{,1..5} (6 alike) : Sin  Amplitude=5  SampleTime=0
  [0...5]{,1..5} (6 alike) : Saturate  UpperLimit=5  LowerLimit=0
  Out1 : Outport
  wires:
  Constant4/1 -> Bus Creator2/3  "brk"
  "[0...5]4"/1 -> Bus Creator2/1  "duty"
  Bus Creator3/1 -> Bus Creator6/1  "tCMD"
  "[0...5]3"/1 -> Bus Creator4/1  "duty"
  Gain4/1 -> Bus Creator2/2  "rev"
  Gain/1 -> Bus Creator3/2  "rev"
  "[0...5]2"/1 -> Bus Creator1/1  "duty"
  Constant/1 -> Bus Creator3/3  "brk"
  Constant2/1 -> Bus Creator1/3  "brk"
  Gain2/1 -> Bus Creator1/2  "rev"
  Gain1/1 -> Bus Creator/2  "rev"
  Constant1/1 -> Bus Creator/3  "brk"
  "[0...5]1"/1 -> Bus Creator/1  "duty"
  Bus Creator4/1 -> Bus Creator6/4  "wCMD"
  "[0...5]"/1 -> Bus Creator3/1  "duty"
  Bus Creator2/1 -> Bus Creator6/5  "hCMD"
  Gain3/1 -> Bus Creator4/2  "rev"
  Bus Creator5/1 -> Bus Creator6/6  "gCMD"
  Constant3/1 -> Bus Creator4/3  "brk"
  Bus Creator1/1 -> Bus Creator6/3  "fCMD"
  Gain5/1 -> Bus Creator5/2  "rev"
  Bus Creator/1 -> Bus Creator6/2  "bCMD"
  Constant5/1 -> Bus Creator5/3  "brk"
  "[0...5]5"/1 -> Bus Creator5/1  "duty"
  Bus Creator6/1 -> Out1/1
  Sine Wave/1 -> Fcn/1, Abs/1
  Fcn/1 -> Gain/1
  Abs/1 -> "[0...5]"/1
  Abs1/1 -> "[0...5]1"/1
  Fcn1/1 -> Gain1/1
  Sine Wave1/1 -> Fcn1/1, Abs1/1
  Abs2/1 -> "[0...5]2"/1
  Sine Wave2/1 -> Abs2/1, Fcn2/1
  Fcn2/1 -> Gain2/1
  Abs3/1 -> "[0...5]3"/1
  Sine Wave3/1 -> Fcn3/1, Abs3/1
  Fcn3/1 -> Gain3/1
  Abs4/1 -> "[0...5]4"/1
  Sine Wave4/1 -> Abs4/1, Fcn4/1
  Fcn4/1 -> Gain4/1
  Abs5/1 -> "[0...5]5"/1
  Sine Wave5/1 -> Abs5/1, Fcn5/1
  Fcn5/1 -> Gain5/1

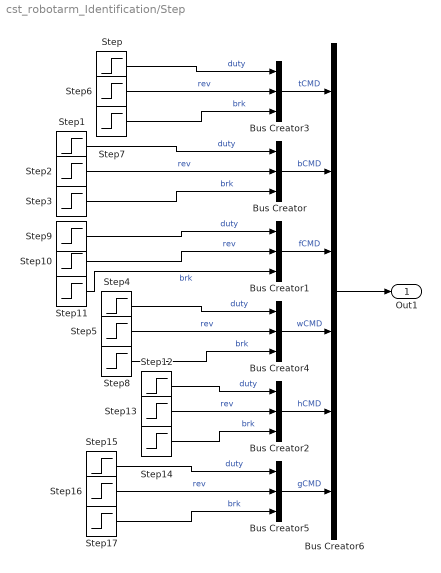
== system cst_robotarm_Identification/Step ==
  Bus Creator{,1..5} (6 alike) : BusCreator  Inputs=3
  Bus Creator6 : BusCreator  Inputs=6
  Step : Step  Time=2  SampleTime=Ts
  Step1 : Step  Time=2  SampleTime=Ts
  Step{2..3,5,7..8,10..11,13..14,16..17} (11 alike) : Step  Time=0  After=0  SampleTime=Ts
  Step12 : Step  Time=20  SampleTime=Ts
  Step15 : Step  Time=25  SampleTime=Ts
  Step4 : Step  Time=15  SampleTime=Ts
  Step6 : Step  Time=0  SampleTime=Ts
  Step9 : Step  Time=10  SampleTime=Ts
  Out1 : Outport
  wires:
  Step14/1 -> Bus Creator2/3  "brk"
  Step12/1 -> Bus Creator2/1  "duty"
  Bus Creator3/1 -> Bus Creator6/1  "tCMD"
  Step4/1 -> Bus Creator4/1  "duty"
  Step13/1 -> Bus Creator2/2  "rev"
  Step6/1 -> Bus Creator3/2  "rev"
  Step9/1 -> Bus Creator1/1  "duty"
  Step7/1 -> Bus Creator3/3  "brk"
  Step11/1 -> Bus Creator1/3  "brk"
  Step10/1 -> Bus Creator1/2  "rev"
  Step2/1 -> Bus Creator/2  "rev"
  Step3/1 -> Bus Creator/3  "brk"
  Step1/1 -> Bus Creator/1  "duty"
  Bus Creator4/1 -> Bus Creator6/4  "wCMD"
  Step/1 -> Bus Creator3/1  "duty"
  Bus Creator2/1 -> Bus Creator6/5  "hCMD"
  Step5/1 -> Bus Creator4/2  "rev"
  Bus Creator5/1 -> Bus Creator6/6  "gCMD"
  Step8/1 -> Bus Creator4/3  "brk"
  Bus Creator1/1 -> Bus Creator6/3  "fCMD"
  Step16/1 -> Bus Creator5/2  "rev"
  Bus Creator/1 -> Bus Creator6/2  "bCMD"
  Step17/1 -> Bus Creator5/3  "brk"
  Step15/1 -> Bus Creator5/1  "duty"
  Bus Creator6/1 -> Out1/1

== system cst_robotarm_Identification/Subsystem3 ==
